simulink model "s_2d_gantry"  (R2025b)
settings: Solver=ode1  StartTime=0.0  StopTime=100  FixedStep=0.002  RelTol=1e-3  EnableMultiTasking=on
undefined symbols (not defined in the file): A, B, C, D, K
libraries: simulink_extras x4, simulink x1
settings Model: SimulationMode=external  ExtModeTrigDuration=10000  Creator=MLevis  LastModifiedBy=USER_NAME
settings SolverCC: AlgebraicLoopSolver=TrustRegion  PositivePriorityOrder=on
settings DataIOCC: LimitDataPoints=on  SaveFormat=Array  SignalLoggingSaveFormat=ModelDataLogs  ReturnWorkspaceOutputs=off
settings OptimizationCC: BooleanDataType=off  OptimizeBlockIOStorage=off  BufferReuse=off  GlobalBufferReuse=off  ExpressionFolding=off  ExpressionDepthLimit=2147483647.0  LocalBlockOutputs=off  InitFltsAndDblsToZero=on
settings DebuggingCC: SaveWithParameterizedLinksMsg=none  UnderspecifiedInitializationDetection=Classic  MergeDetectMultiDrivingBlocksExec=none  SignalResolutionControl=TryResolveAllWithWarning  MultiTaskDSMMsg=warning  MultiTaskCondExecSysMsg=none  FcnCallInpInsideContextMsg=warning  UnconnectedInputMsg=warning  UnconnectedOutputMsg=warning  UnconnectedLineMsg=warning  StateNameClashWarn=warning  SFUnexpectedBacktrackingDiag=warning  SFNoUnconditionalDefaultTransitionDiag=warning  SFExecutionAtInitializationDiag=none  ArithmeticOperatorsInVariantConditions=warning
settings HardwareCC: ProdBitPerPointer=32.0  ProdBitPerSizeT=32.0  ProdBitPerPtrDiffT=32.0  ProdLargestAtomicFloat=None  ProdIntDivRoundTo=Undefined  ProdEndianess=Unspecified  ProdWordSize=32.0  ProdHWDeviceType=32-bit Generic  TargetHWDeviceType=32-bit Generic
settings ModelReferenceCC: EnableRefExpFcnMdlSchedulingChecks=on  PropagateSignalLabelsOutOfModel=off
settings SFSimCC: SimUseLocalCustomCode=off  CustomCodeUndefinedFunction=UseInterfaceOnly
settings RTWCC: SystemTargetFile=quarc_win64.tlc  TemplateMakefile=quarc_default_tmf  RTWUseLocalCustomCode=off  GPUComputeCapability=3.5  Description=QUARC Win64 Target
settings CodeAppCC: StateflowObjectComments=on
settings STFCustomTargetCC: SystemTargetFile=quarc_win64.tlc  TargetPreCompLibLocation=C:\PROGRA~3\QUARC\lib\2016b\win64\release  StopOnOverrun=off  DownloadToTarget=on  Debug=off
settings GRTTargetCC: ExtMode=on  ExtModeMexFile=quarc_comm  TargetPreCompLibLocation=C:\PROGRA~3\QUARC\lib\2016b\win64\release  TargetLangStandard=C89/C90 (ANSI)  ParMdlRefBuildCompliant=off  CompOptLevelCompliant=off  CombineOutputUpdateFcns=off  MatFileLogging=off  CPPClassGenCompliant=off  GRTInterface=on  UseToolchainInfoCompliant=off
settings ConfigComp: CovMetricSettings=dw  CovSaveCumulativeToWorkspaceVar=on  CovSaveSingleToWorkspaceVar=on  CovExternalEMLEnable=off

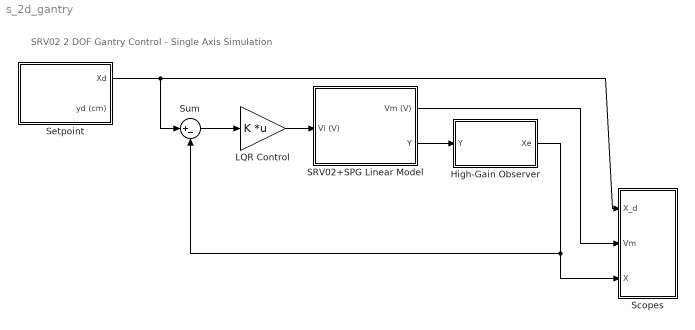
== system s_2d_gantry ==
  note: SRV02 2 DOF Gantry Control - Single Axis Simulation
  High-Gain Observer : Subsystem
  LQR Control : Gain  Gain=K  Multiplication=Matrix(K*u)  SaturateOnIntegerOverflow=on  OutDataTypeStr=Inherit: Same as input  ParamDataTypeStr=Inherit: Same as input
  SRV02+SPG Linear Model : Subsystem
  Scopes : Subsystem
  Setpoint : Subsystem
  Sum : Sum  Inputs=|+-
  wires:
  Setpoint/1(Xd) -> Sum/1, Scopes/1(X_d)
  High-Gain Observer/1(Xe) -> Sum/2, Scopes/3(X)
  SRV02+SPG Linear Model/1(Vm (V)) -> Scopes/2(Vm)
  SRV02+SPG Linear Model/2(Y) -> High-Gain Observer/1(Y)
  LQR Control/1 -> SRV02+SPG Linear Model/1(Vi (V))
  Sum/1 -> LQR Control/1

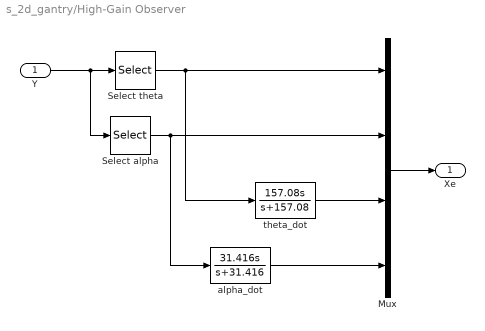
== system s_2d_gantry/High-Gain Observer ==
  Y : Inport
  Mux : Mux
  Select alpha : Selector  InputPortWidth=2  IndexOptions=Index vector (dialog)  Indices=2  OutputSizes=1
  Select theta : Selector  InputPortWidth=2  IndexOptions=Index vector (dialog)  Indices=1  OutputSizes=1
  alpha_dot : TransferFcn  Numerator=[31.416 0]  Denominator=[1 31.416]
  theta_dot : TransferFcn  Numerator=[157.08 0]  Denominator=[1 157.08]
  Xe : Outport
  wires:
  Select alpha/1 -> alpha_dot/1, Mux/2
  Mux/1 -> Xe/1
  Y/1 -> Select alpha/1, Select theta/1
  theta_dot/1 -> Mux/3
  Select theta/1 -> theta_dot/1, Mux/1
  alpha_dot/1 -> Mux/4

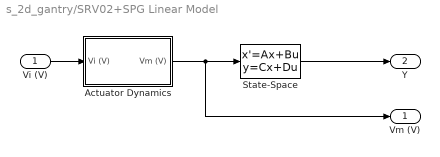
== system s_2d_gantry/SRV02+SPG Linear Model ==
  Vi (V) : Inport
  Actuator Dynamics : Subsystem
  State-Space : StateSpace  A=A  B=B  C=C  D=D  InitialCondition=0
  Vm (V) : Outport
  Y : Outport  Port=2
  wires:
  State-Space/1 -> Y/1
  Vi (V)/1 -> Actuator Dynamics/1(Vi (V))
  Actuator Dynamics/1(Vm (V)) -> State-Space/1, Vm (V)/1

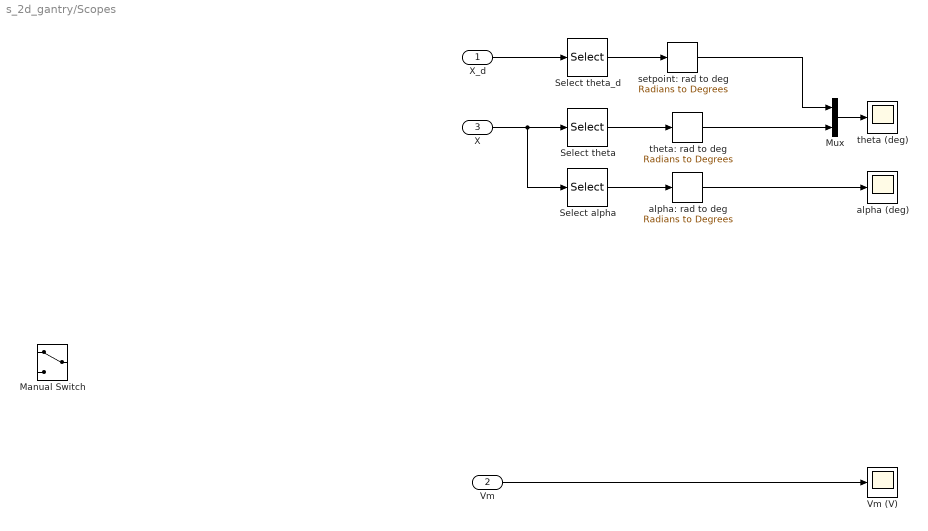
== system s_2d_gantry/Scopes ==
  X_d : Inport
  Vm : Inport  Port=2
  X : Inport  Port=3
  Manual Switch : ManualSwitch
  Mux : Mux  Inputs=2
  Select alpha : Selector  InputPortWidth=4  IndexOptions=Index vector (dialog)  Indices=2  OutputSizes=1
  Select theta : Selector  InputPortWidth=4  IndexOptions=Index vector (dialog)  Indices=1  OutputSizes=1
  Select theta_d : Selector  InputPortWidth=4  IndexOptions=Index vector (dialog)  Indices=1  OutputSizes=1
  Vm (V) : Scope
      settings: TimeSpan=50  ActiveDisplayYMinimum=-18.75  ActiveDisplayYMaximum=18.75  DataLoggingVariableName=data_vm  DataLoggingSaveFormat=Array
  alpha (deg) : Scope
      settings: TimeSpan=50  ActiveDisplayYMinimum=-16.759949348082646  ActiveDisplayYMaximum=16.705844619606239  DataLoggingVariableName=data_alpha  DataLoggingSaveFormat=Array
  alpha: rad to deg : simulink_extras/Transformations/Radians to Degrees
  setpoint: rad to deg : simulink_extras/Transformations/Radians to Degrees
  theta (deg) : Scope
      settings: TimeSpan=50  ActiveDisplayYMinimum=-59.436469905760752  ActiveDisplayYMaximum=64.660837616407377  DataLoggingVariableName=data_theta  DataLoggingSaveFormat=Array
  theta: rad to deg : simulink_extras/Transformations/Radians to Degrees
  wires:
  Select theta_d/1 -> setpoint: rad to deg/1
  setpoint: rad to deg/1 -> Mux/1
  X/1 -> Select alpha/1, Select theta/1
  alpha: rad to deg/1 -> alpha (deg)/1
  Select theta/1 -> theta: rad to deg/1
  Select alpha/1 -> alpha: rad to deg/1
  theta: rad to deg/1 -> Mux/2
  Mux/1 -> theta (deg)/1
  X_d/1 -> Select theta_d/1
  Vm/1 -> Vm (V)/1

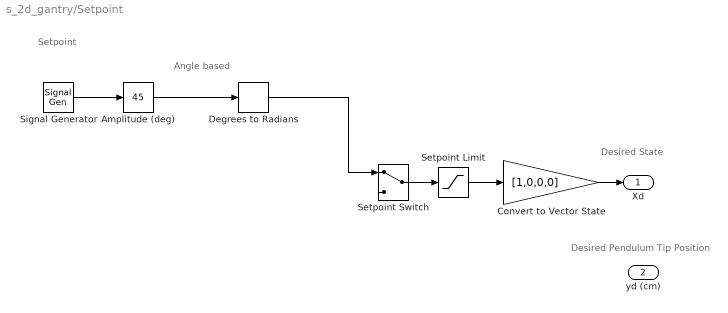
== system s_2d_gantry/Setpoint ==
  note: Angle based
  note: Setpoint
  note: Desired State
  note: Desired Pendulum Tip Position
  Amplitude (deg) : simulink/Math Operations/Slider Gain  gain=45  low=0  high=75
  Convert to Vector State : Gain  Gain=[1,0,0,0]
  Degrees to Radians : simulink_extras/Transformations/Degrees to Radians
  Setpoint Switch : ManualSwitch
  Setpoint Limit : Saturate  UpperLimit=15  LowerLimit=-15
  Signal Generator : SignalGenerator  WaveForm=square  Frequency=0.05
  Xd : Outport
  yd (cm) : Outport  Port=2
  wires:
  Setpoint Limit/1 -> Convert to Vector State/1
  Convert to Vector State/1 -> Xd/1
  Setpoint Switch/1 -> Setpoint Limit/1
  Degrees to Radians/1 -> Setpoint Switch/1
  Signal Generator/1 -> Amplitude (deg)/1
  Amplitude (deg)/1 -> Degrees to Radians/1

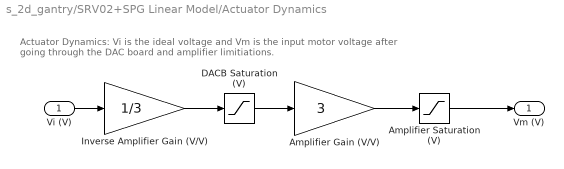
== system s_2d_gantry/SRV02+SPG Linear Model/Actuator Dynamics ==
  note: Actuator Dynamics: Vi is the ideal voltage and Vm is the
      | input motor voltage after going through the DAC board and amplifier limitiations.
  Vi (V) : Inport
  Amplifier Gain (V/V) : Gain  Gain=3
  Amplifier Saturation (V) : Saturate  UpperLimit=15  LowerLimit=-15
  DACB Saturation (V) : Saturate  UpperLimit=15  LowerLimit=-15
  Inverse Amplifier Gain (V/V) : Gain  Gain=1/3
  Vm (V) : Outport
  wires:
  Inverse Amplifier Gain (V/V)/1 -> DACB Saturation (V)/1
  DACB Saturation (V)/1 -> Amplifier Gain (V/V)/1
  Amplifier Gain (V/V)/1 -> Amplifier Saturation (V)/1
  Vi (V)/1 -> Inverse Amplifier Gain (V/V)/1
  Amplifier Saturation (V)/1 -> Vm (V)/1
